simulink model "factory"  (R2023a)
settings: Solver=FixedStepDiscrete  StartTime=0.0  StopTime=inf  RelTol=1e-3
values from neighbouring files (symbols this model uses):
  A_discrete = A_cont*dt_kf+eye(4)    [perceptionsetup.m]
  C = [1 0 0 0;0 1 0 0]    [perceptionsetup.m]
  dt_control = 0.010    (= 0.01)    [start.m]
  dt_kf = 0.040    (= 0.04)    [perceptionsetup.m]
  dt_predictor = 0.010    (= 0.01)    [perceptionsetup.m]
  Q = dt_kf^2*diag([xDot_err_var, xDot_err_var, vxDot_err_var, vxDot_err_var])    [perceptionsetup.m]
  Qbad = dt_kf^2*diag([1 1 1 1])    [perceptionsetup.m]
  R = 2.5e-5*diag([1 1])    [perceptionsetup.m]
undefined symbols (not defined in the file or in its folder): Discrete, Time
libraries: simulink x4, visionsinks x2, mjLib x2, ctrlSharedLib x1, visiontextngfix x1
settings Model: NumberOfSteps=40  Creator=vmano  LastModifiedBy=vmano
settings OptimizationCC: ReuseModelBlockBuffer=off  ZeroExternalMemoryAtStartup=off  ZeroInternalMemoryAtStartup=off
settings HardwareCC: ProdHWDeviceType=AMD->x86-64 (Windows64)
settings SFSimCC: SimTargetLang=C++
settings RTWCC: TargetLang=C++
settings GRTTargetCC: TargetLangStandard=C++11 (ISO)  CodeInterfacePackaging=C++ class

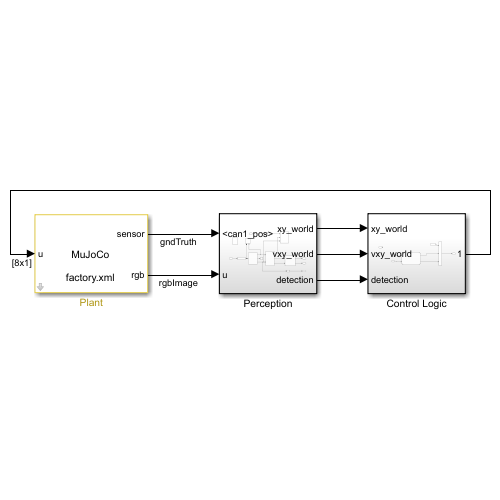
[thumbnail: Simulink's stored preview of the top-level diagram]
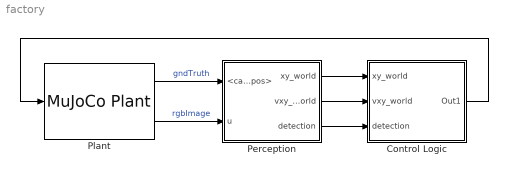
== system factory ==
  Control Logic : Subsystem
  Perception : Subsystem
  Plant : mjLib/MuJoCo Plant  controlBus=[]  sensorBus=mj_bus_sensor_7979902499018342666  controlLength=[]  sensorLength=[]  rgbLength=[]  depthLength=[]  sampleTime=0.001  xmlFileRel=factory.xml  xmlFile=D:\manoj_stuff\mujoco-demo\examples\models\factory.xml  renderingType=Global  vsync=off  visualFPS=60  zoomLevel=1  znear=0.03  zfar=150  cameraSampleTime=dt_kf  rgbOutOption=on  depthOutOption=off  controlInterfaceType=Vector
      settings: SourceProductName=MuJoCo Simulator
  wires:
  Control Logic/1(Out1) -> Plant/1
  Plant/1 -> Perception/1(<can1_pos>)  "gndTruth"
  Plant/2 -> Perception/2(u)  "rgbImage"
  Perception/1(xy_world) -> Control Logic/1(xy_world)
  Perception/2(vxy_world) -> Control Logic/2(vxy_world)
  Perception/3(detection) -> Control Logic/3(detection)

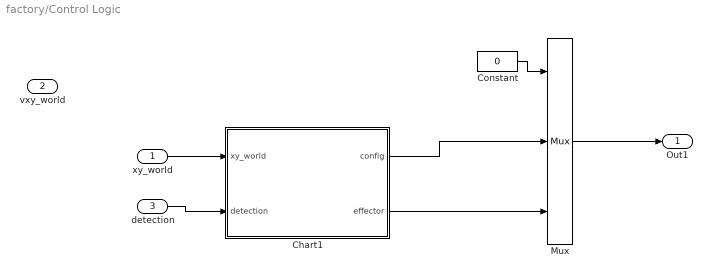
== system factory/Control Logic ==
  xy_world : Inport
  vxy_world : Inport  Port=2
  detection : Inport  Port=3
  Chart1 : Stateflow chart  InitFcn=clear planner  TreatAsAtomicUnit=on  SystemSampleTime=dt_control
      settings: PortSchema="{\"entries\":[{\"content\":{\"sides\":[{\"content\":{\"connectorIds\":[\"In1\",\"In2\"]},\"type\":\"ConnectorPlacement.EquallySpacedRectSide\",\"uuid\":\"afb73485-7f81-405a-bce0-f65bd38353b1\"},{\"content\":{\"connectorIds\":[\"Out2\",\"Out1\"],\"side\":\"RIGHT\"},\"type\":\"ConnectorPlacement.EquallySpacedRectSide\",\"uuid\":\"632edaa2-b5d3-4885-8368-fb2a3f139835\"},{\"content\":{\"side\":\"TOP\"},\"type\":\"ConnectorPlacement.EquallySpacedRectSide\",\"uuid\":\"25e57255-c002-4900-a084-700ea23880f8\"}]},\"type\":\"ConnectorPlacement.EquallySpacedConnector\",\"uuid\":\"861ccd4d-a85c-4c22-af63-d1b2e3344d54\"}],\"packageUris\":[\"http://schema.mathworks.com/mf0/Connector/R2020b\"],\"version\":\"1.0\"}"
  Constant : Constant  Value=0
  Mux : Mux  Inputs=3
  Out1 : Outport
  wires:
  xy_world/1 -> Chart1/1(xy_world)
  Mux/1 -> Out1/1
  Chart1/2(config) -> Mux/2
  Chart1/1(effector) -> Mux/3
  detection/1 -> Chart1/2(detection)
  Constant/1 -> Mux/1

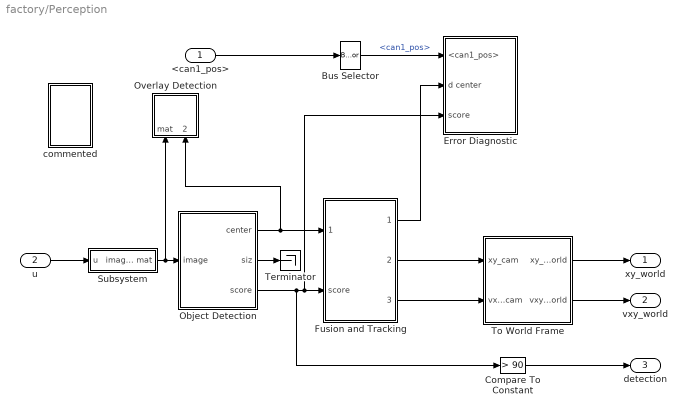
== system factory/Perception ==
  <can1_pos> : Inport
  u : Inport  Port=2
  Bus Selector : BusSelector  OutputSignals=can1_pos
  Compare To Constant : simulink/Logic and Bit Operations/Compare To Constant  relop=>  const=90  OutDataTypeStr=boolean
  Error Diagnostic : Subsystem
  Fusion and Tracking : Subsystem
  Object Detection : MATLAB Function  TreatAsAtomicUnit=on
  Overlay Detection : Subsystem
  Subsystem : Subsystem
  Terminator : Terminator
  To World Frame : Subsystem
  commented : Subsystem
  xy_world : Outport
  vxy_world : Outport  Port=2
  detection : Outport  Port=3
  wires:
  Object Detection/3(score) -> Compare To Constant/1, Fusion and Tracking/2(score), Error Diagnostic/3(score)
  Subsystem/1(image mat) -> Overlay Detection/1(mat), Object Detection/1(image)
  Fusion and Tracking/2(xy_camKF) -> To World Frame/1(xy_cam)
  Fusion and Tracking/3(vxy_camKF) -> To World Frame/2(vxy_cam)
  u/1 -> Subsystem/1(u)
  To World Frame/1(xy_world) -> xy_world/1
  To World Frame/2(vxy_world) -> vxy_world/1
  <can1_pos>/1 -> Bus Selector/1
  Object Detection/1(center) -> Fusion and Tracking/1(xy_pixel), Overlay Detection/2(center)
  Object Detection/2(siz) -> Terminator/1
  Bus Selector/1 -> Error Diagnostic/1(<can1_pos>)  "<can1_pos>"
  Fusion and Tracking/1(xy_camRaw) -> Error Diagnostic/2(d center)
  Compare To Constant/1 -> detection/1

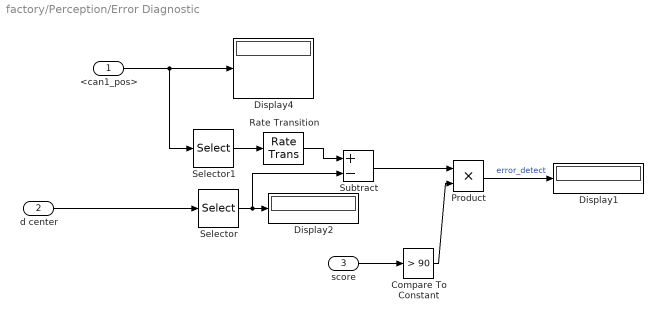
== system factory/Perception/Error Diagnostic ==
  <can1_pos> : Inport
  d center : Inport  Port=2
  score : Inport  Port=3
  Compare To Constant : simulink/Logic and Bit Operations/Compare To Constant  relop=>  const=90  OutDataTypeStr=boolean
  Display1 : Display
  Display2 : Display
  Display4 : Display
  Product : Product
  Rate Transition : RateTransition
  Selector : Selector  IndexOptions=Index vector (dialog)  Indices=[1]  OutputSizes=1
  Selector1 : Selector  IndexOptions=Index vector (dialog)  Indices=2  OutputSizes=1
  Subtract : Sum  Inputs=+-
  wires:
  Selector/1 -> Subtract/2, Display2/1
  d center/1 -> Selector/1
  Rate Transition/1 -> Subtract/1
  <can1_pos>/1 -> Display4/1, Selector1/1
  Subtract/1 -> Product/1
  Selector1/1 -> Rate Transition/1
  Product/1 -> Display1/1  "error_detect"
  Compare To Constant/1 -> Product/2
  score/1 -> Compare To Constant/1

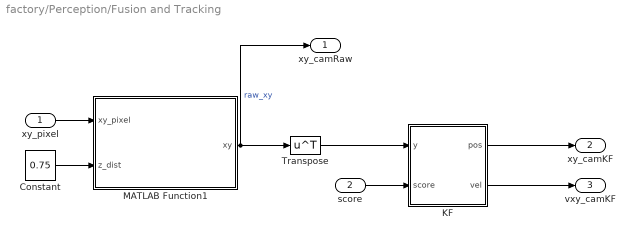
== system factory/Perception/Fusion and Tracking ==
  xy_pixel : Inport
  score : Inport  Port=2
  Constant : Constant  Value=0.75
  KF : Subsystem
  MATLAB Function1 : MATLAB Function  TreatAsAtomicUnit=on
  Transpose : Math  Operator=transpose
  xy_camRaw : Outport
  xy_camKF : Outport  Port=2
  vxy_camKF : Outport  Port=3
  wires:
  xy_pixel/1 -> MATLAB Function1/1(xy_pixel)
  score/1 -> KF/2(score)
  Constant/1 -> MATLAB Function1/2(z_dist)
  Transpose/1 -> KF/1(y)
  MATLAB Function1/1(xy) -> xy_camRaw/1, Transpose/1  "raw_xy"
  KF/1(pos) -> xy_camKF/1
  KF/2(vel) -> vxy_camKF/1

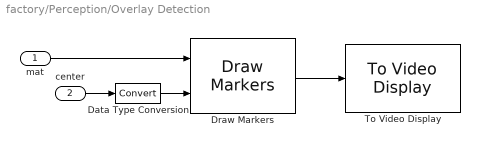
== system factory/Perception/Overlay Detection ==
  mat : Inport
  center : Inport  Port=2
  Data Type Conversion : DataTypeConversion  SaturateOnIntegerOverflow=off  RndMeth=Floor
  Draw Markers : visiontextngfix/Draw Markers  shape=Circle  size=10  fill=on  fillClrSource=Specify via dialog  display=Black  intensity=200  color=[200 255 100]  opacity=0.6  viewport=Entire image  antialiasing=on  inType=Obsolete  imagePorts=One multidimensional signal  roundingMode=Floor  overflowMode=off  memoryMode=Specify word length  memoryWordLength=16  memoryFracLength=15  prodOutputMode=Binary point scaling  prodOutputWordLength=32  prodOutputFracLength=14
  To Video Display : visionsinks/To Video Display  windowSizeMode=Normal  openAtMdlStart=on  fullScreen=off  videoWindowX=1099  videoWindowY=111  saveWindowSize=off  videoWindowWidth=698  videoWindowHeight=368  inputColorFormat=RGB  inputType=Obsolete  imagePorts=One multidimensional signal  OutputDevice=On-screen video monitor  dataOrg=Column-major  isWindowOpen=off
  wires:
  Draw Markers/1 -> To Video Display/1
  mat/1 -> Draw Markers/1
  center/1 -> Data Type Conversion/1
  Data Type Conversion/1 -> Draw Markers/2

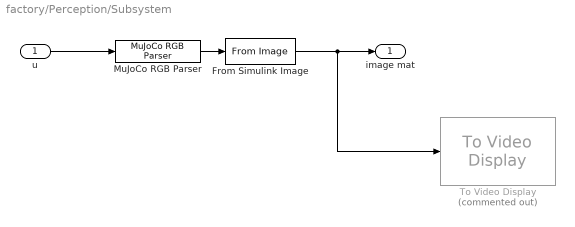
== system factory/Perception/Subsystem ==
  u : Inport
  From Simulink Image : FromImage
  MuJoCo RGB Parser : mjLib/MuJoCo RGB Parser  inputBusType=mj_bus_rgb_6905886718754851708  selectedCamera=rgbcam  imageRows=480  imageCols=640  startingIndex=1  endingIndex=921600
      settings: SourceProductName=MuJoCo Simulator
  To Video Display : visionsinks/To Video Display  Commented=on  windowSizeMode=Normal  openAtMdlStart=on  fullScreen=off  videoWindowX=536805376  videoWindowY=536805376  saveWindowSize=off  videoWindowWidth=640  videoWindowHeight=480  inputColorFormat=RGB  inputType=Obsolete  imagePorts=One multidimensional signal  OutputDevice=On-screen video monitor  dataOrg=Column-major  isWindowOpen=off
  image mat : Outport
  wires:
  MuJoCo RGB Parser/1 -> From Simulink Image/1
  u/1 -> MuJoCo RGB Parser/1
  From Simulink Image/1 -> To Video Display/1, image mat/1

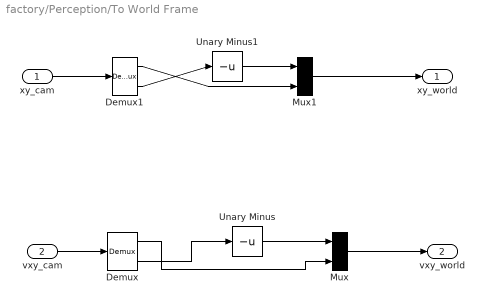
== system factory/Perception/To World Frame ==
  xy_cam : Inport
  vxy_cam : Inport  Port=2
  Demux : Demux  Outputs=2
  Demux1 : Demux  Outputs=2
  Mux : Mux  Inputs=2
  Mux1 : Mux  Inputs=2
  Unary Minus : UnaryMinus
  Unary Minus1 : UnaryMinus
  xy_world : Outport
  vxy_world : Outport  Port=2
  wires:
  Mux/1 -> vxy_world/1
  vxy_cam/1 -> Demux/1
  Demux/1 -> Mux/2
  Unary Minus/1 -> Mux/1
  Demux/2 -> Unary Minus/1
  xy_cam/1 -> Demux1/1
  Mux1/1 -> xy_world/1
  Demux1/1 -> Mux1/2
  Unary Minus1/1 -> Mux1/1
  Demux1/2 -> Unary Minus1/1

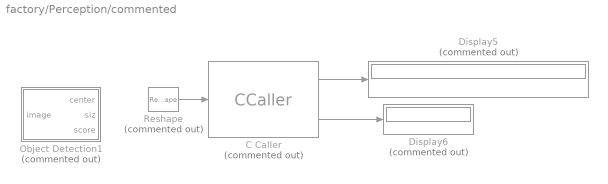
== system factory/Perception/commented ==
  C Caller : CCaller  Commented=on  FunctionName=slDetect  PortSpecificationStruct="%)30     .    @ 4   8    (     @         %    \"     ,    !     0         %  0 \"0    $    _    07)G3F%M90  4&]R=$YA;64 4V-O<&4     26YD97@     5'EP90      4VEZ90      27-';&]B86P   X    X    !@    @    $          4    (     0    4    !         !     %    :6UA9V4    .    .     8    (    !          %    \"     $    %     0         0    !0   &EM86=E    #@   #@    &    \"     0         !0    @    !    !0    $         $     4   !);G!U=     X    X    !@    @    &          4    (     0    $    !          D    (               .    .     8    (    !          %    \"     $    %     0         0    !0   '5I;G0X    #@   #@    &    \"     0         !0    @    !    !@    $         $     8    Y,C$V,#    X    P    !@    @    ) @        4    (     0    $    !          (  0      #@   #     &    \"     0         !0    @    !    !     $         $  $ &)B;W@.    ,     8    (    !          %    \"     $    $     0         0  0 8F)O> X    X    !@    @    $          4    (     0    8    !         !     &    3W5T<'5T   .    .     8    (    !@         %    \"     $    !     0         )    \"               #@   #@    &    \"     0         !0    @    !    !@    $         $     8   !D;W5B;&4   X    P    !@    @    $          4    (     0    $    !         !   0 T    #@   #     &    \"     D\"        !0    @    !     0    $          @ !       .    .     8    (    !          %    \"     $    %     0         0    !0   '-C;W)E    #@   #@    &    \"     0         !0    @    !    !0    $         $     4   !S8V]R90    X    X    !@    @    $          4    (     0    8    !         !     &    3W5T<'5T   .    .     8    (    !@         %    \"     $    !     0         )    \"            / _#@   #@    &    \"     0         !0    @    !    !@    $         $     8   !D;W5B;&4   X    P    !@    @    $          4    (     0    $    !         !   0 Q    #@   #     &    \"     D\"        !0    @    !     0    $          @ !"
  Display5 : Display  Commented=on
  Display6 : Display  Commented=on
  Object Detection1 : MATLAB Function  Commented=on  TreatAsAtomicUnit=on
  Reshape : Reshape  Commented=on
  wires:
  C Caller/1 -> Display5/1
  C Caller/2 -> Display6/1
  Reshape/1 -> C Caller/1

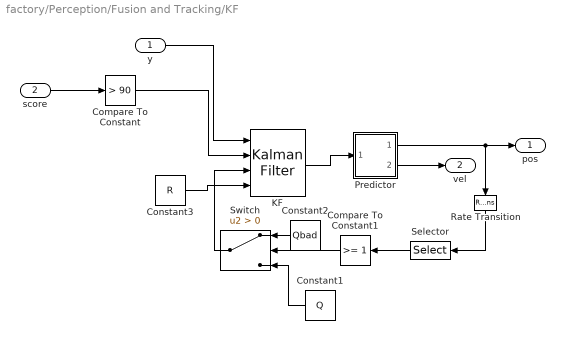
== system factory/Perception/Fusion and Tracking/KF ==
  y : Inport
  score : Inport  Port=2
  Compare To Constant : simulink/Logic and Bit Operations/Compare To Constant  relop=>  const=90  OutDataTypeStr=boolean
  Compare To Constant1 : simulink/Logic and Bit Operations/Compare To Constant  relop=>=  const=1  OutDataTypeStr=boolean
  Constant1 : Constant  Value=Q
  Constant2 : Constant  Value=Qbad
  Constant3 : Constant  Value=R
  KF : ctrlSharedLib/Kalman Filter  TimeDomain=Discrete-Time  UseCurrentEstimator=on  ModelSource=Individual A, B, C, D matrices  ModelSourceVariable=ss(0.95,1,1,0,1)  A=A_discrete  B=1  C=C  D=0  NumberOfStates=1  NumberOfInputs=1  NumberOfOutputs=1  InitialEstimateSource=Dialog  X0=0  P0=P0  UseK=off  UseGH=off  NumberOfProcessNoiseInputs=1  G=1  TimeInvariantG=on  H=0  TimeInvariantH=on  Q=Q  TimeInvariantQ=off  R=R  TimeInvariantR=off  N=0  TimeInvariantN=on  AddInputPort=off  AddEnablePort=on  OutputEstimatedY=off  OutputP=off  Ts=dt_kf
  Predictor : Subsystem
  Rate Transition : RateTransition
  Selector : Selector  IndexOptions=Index vector (dialog)  Indices=2  OutputSizes=1
  Switch : Switch  Criteria=u2 > Threshold  SaturateOnIntegerOverflow=off  InputSameDT=off
  pos : Outport
  vel : Outport  Port=2
  wires:
  y/1 -> KF/1
  score/1 -> Compare To Constant/1
  Compare To Constant/1 -> KF/2
  Predictor/1(Out1) -> Rate Transition/1, pos/1
  Predictor/2(Out2) -> vel/1
  Constant3/1 -> KF/4
  KF/1 -> Predictor/1(x_s)
  Selector/1 -> Compare To Constant1/1
  Rate Transition/1 -> Selector/1
  Compare To Constant1/1 -> Switch/2
  Constant1/1 -> Switch/3
  Switch/1 -> KF/3
  Constant2/1 -> Switch/1

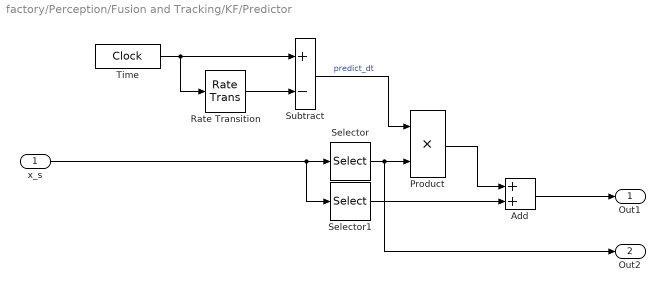
== system factory/Perception/Fusion and Tracking/KF/Predictor ==
  x_s : Inport
  Add : Sum
  Product : Product
  Rate Transition : RateTransition  OutPortSampleTime=dt_kf
  Selector : Selector  IndexOptions=Index vector (dialog)  Indices=[3 4]  OutputSizes=1
  Selector1 : Selector  IndexOptions=Index vector (dialog)  Indices=[1 2]  OutputSizes=1
  Subtract : Sum  Inputs=+-
  Time : DigitalClock  SampleTime=dt_predictor
  Out1 : Outport
  Out2 : Outport  Port=2
  wires:
  Time/1 -> Subtract/1, Rate Transition/1
  Subtract/1 -> Product/1  "predict_dt"
  Add/1 -> Out1/1
  Rate Transition/1 -> Subtract/2
  Selector/1 -> Out2/1, Product/2
  x_s/1 -> Selector1/1, Selector/1
  Product/1 -> Add/1
  Selector1/1 -> Add/2

== stateflow chart factory/Control Logic/Chart1 ==
  state PLANNING
    en:
    coder.extrinsic('planner');
    [jointTraj, timesamples, N] = planner(goalXYZ);
    index = 1;
  state PICK
    en, du:
    if abs(xy_world(2)-1)<0.005
    effector = 20;
    goalXYZ(3) = 0.8;
    transition = true;
    task = 1;
    end
  state SEND_WP
    en:
    config = jointTraj(index, 1:6)';
    index = index+1;
  state SET_PLACE_XYZ
    en:
    goalXYZ = dropSite;
    transition = true;
    task =3;
  state WAIT
    en:
  state DROP
    en:
    effector = 0;
    dropSite = dropSite+[-0.0355 0 0];
  state SET_NEXT_PICK_XYZ
    en:
    du:
    if detection && xy_world(2)>0
    transition = true;
    task = 0;
    pickSite = [xy_world(1) 1 0.716];
    goalXYZ = pickSite;
    end
  (junction 58) -> PLANNING
  (junction 46) -> (junction 58) : [transition]{transition=false}
  PLANNING -> SEND_WP
  PICK -> (junction 46)
  (junction 43) -> PICK [order 1] : [task == 0]
  SEND_WP -> SEND_WP [order 2] : [after(plannerTimeStep, sec)]
  SEND_WP -> WAIT [order 1] : [index>6]
  SET_PLACE_XYZ -> (junction 46)
  SET_NEXT_PICK_XYZ -> (junction 46)
  WAIT -> (junction 43) : [after(2*plannerTimeStep, sec)]
  (junction 43) -> SET_PLACE_XYZ [order 2] : [task == 1]
  (junction 43) -> DROP [order 3] : [task == 3]
  (default) -> SET_NEXT_PICK_XYZ
  DROP -> SET_NEXT_PICK_XYZ : [after(0.4, sec)]
  data: effector output =0; config output =zeros(6,1); jointTraj local; index local; goalXYZ local =[0, 1 , 0.722]; xy_world input; plannerTimeStep constant double =plannerTimeStep; transition local =false; task local =0; dropSite local = [-0.435 0.735 0.85]; pickSite local; detection input; timesamples local; N local

== matlab function factory/Perception/Fusion and Tracking/MATLAB Function1 ==
  data: xy_pixel input; xy output; z_dist input
function xy = toCamCoord(xy_pixel, z_dist)

fovy = 48.8;
camres = [640 480];

% pin hole camera model
focal_pixels = 0.5*camres(2)/tand(fovy/2);

xy = z_dist*((xy_pixel-camres*0.5)/focal_pixels);

== matlab function factory/Perception/Object Detection ==
  data: image input; center output; siz output; score output
function [center, siz, score] = fcn(image)


coder.extrinsic('slDetect_mex');

bbox = zeros(1, 4);
score = 0;
[bbox, score] = slDetect_mex(image);

siz = bbox(3:4);
center = bbox(1:2)+siz*0.5;


end

== matlab function factory/Perception/commented/Object Detection1 ==
  data: image input; center output; siz output; score output
function [center, siz, score] = fcn(image)


coder.extrinsic('slDetect');

bbox = zeros(1, 4);
score = 0;
[bbox, score] = slDetect(image);

siz = bbox(3:4);
center = bbox(1:2)+siz/2;


end
